simulink model "model1v2"  (R2020b)
settings: Solver=VariableStepAuto  StartTime=0.0  StopTime=30.0  RelTol=1e-3
settings Model: Creator=dkravchenko  LastModifiedBy=dkravchenko

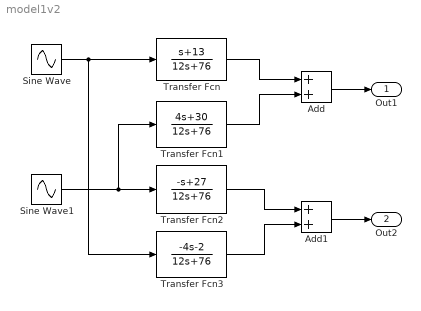
== system model1v2 ==
  Add : Sum
  Add1 : Sum
  Sine Wave : Sin  Amplitude=0  Bias=1  SampleTime=0
  Sine Wave1 : Sin  Amplitude=2  SampleTime=0
  Transfer Fcn : TransferFcn  Numerator=[1 13]  Denominator=[12 76]
  Transfer Fcn1 : TransferFcn  Numerator=[4 30]  Denominator=[12 76]
  Transfer Fcn2 : TransferFcn  Numerator=[-1 27]  Denominator=[12 76]
  Transfer Fcn3 : TransferFcn  Numerator=[-4 -2]  Denominator=[12 76]
  Out1 : Outport
  Out2 : Outport  Port=2
  wires:
  Sine Wave/1 -> Transfer Fcn3/1, Transfer Fcn/1
  Sine Wave1/1 -> Transfer Fcn1/1, Transfer Fcn2/1
  Transfer Fcn/1 -> Add/1
  Transfer Fcn1/1 -> Add/2
  Transfer Fcn2/1 -> Add1/1
  Transfer Fcn3/1 -> Add1/2
  Add/1 -> Out1/1
  Add1/1 -> Out2/1
